simulink model "Question_2"  (R2024b)
settings: Solver=VariableStepAuto  StartTime=0.0  StopTime=10.0  RelTol=1e-3
settings Model: Creator=Sagar  LastModifiedBy=Sagar

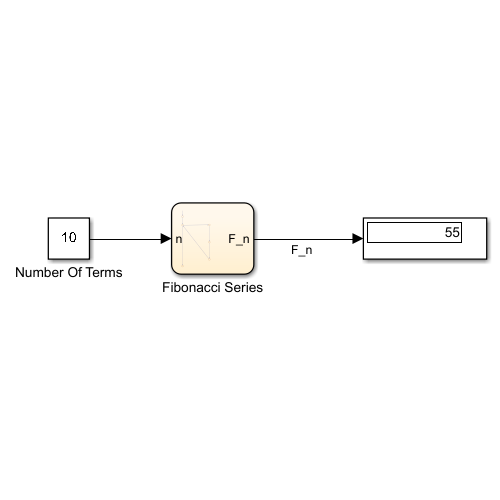
[thumbnail: Simulink's stored preview of the top-level diagram]
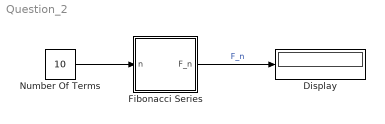
== system Question_2 ==
  Display : Display
  Fibonacci Series : Stateflow chart  TreatAsAtomicUnit=on
  Number Of Terms : Constant  Value=10
  wires:
  Number Of Terms/1 -> Fibonacci Series/1(n)
  Fibonacci Series/1(F_n) -> Display/1  "F_n"

== stateflow chart Question_2/Fibonacci Series ==
  (default) -> (junction 21) : % Fibonacci series
  (junction 21) -> (junction 23) : {i=3;F_n_2=1;F_n_1=1}
  (junction 23) -> (junction 22) [order 1] : [i<=n]
  (junction 22) -> (junction 24) : {F_n=F_n_2+F_n_1;F_n_2=F_n_1;F_n_1=F_n;}
  (junction 25) -> (junction 23)
  (junction 23) -> (junction 26) [order 2]
  (junction 24) -> (junction 25) : {i = i + 1;}
  data: n input; F_n_2 local; F_n_1 local; i local; F_n output
